simulink model "discreteMod2"  (R2019b)
settings: Solver=VariableStepAuto  StartTime=0.0  StopTime=10.0  RelTol=1e-3
settings Model: Creator=Daniel  LastModifiedBy=Daniel

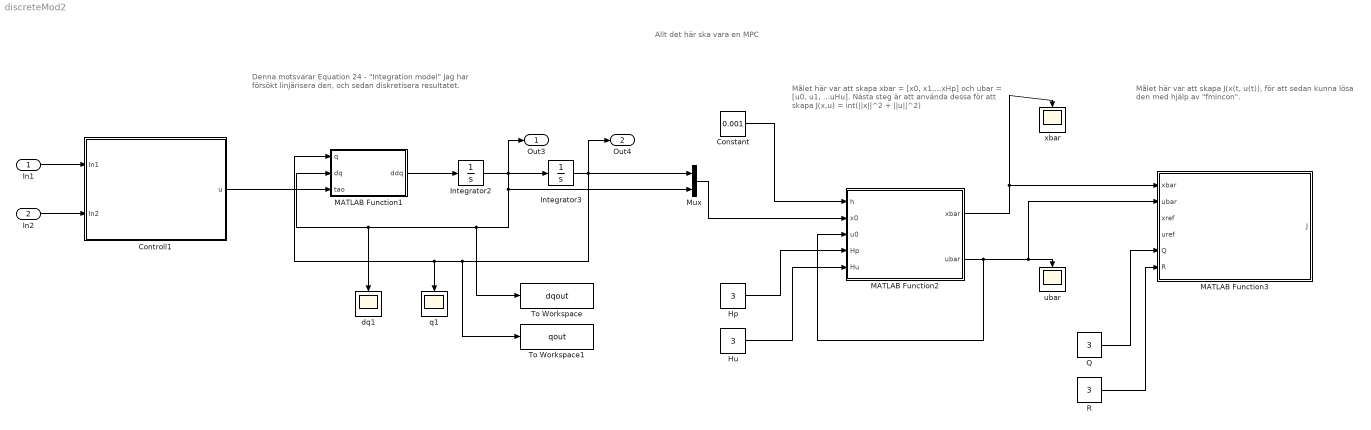
== system discreteMod2 ==
  note: Allt det här ska vara en MPC
  note: Målet här var att skapa J(x(t, u(t)), för att sedan
      | kunna lösa den med hjälp av "fmincon".
  note: Målet här var att skapa xbar = [x0, x1,...xHp]
      | och ubar = [u0, u1, ...uHu].
      | Nästa steg är att använda dessa för att skapa
      | J(x,u) = int(||x||^2 + ||u||^2)
  note: Denna motsvarar
      | Equation 24 - "Integration model"
      | Jag har försökt linjärisera den, och sedan
      | diskretisera resultatet.
  In1 : Inport
  In2 : Inport  Port=2
  Constant : Constant  Value=0.001
  Controll1 : Subsystem
  "Hp " : Constant  Value=3
  "Hu " : Constant  Value=3
  Integrator2 : Integrator  InitialCondition=[0;pi/6]
  Integrator3 : Integrator  InitialCondition=[0;0]
  MATLAB Function1 : MATLAB Function  TreatAsAtomicUnit=on
  MATLAB Function2 : MATLAB Function  TreatAsAtomicUnit=on
  MATLAB Function3 : MATLAB Function  TreatAsAtomicUnit=on
  Mux : Mux  Inputs=2
  Q : Constant  Value=3
  R : Constant  Value=3
  To Workspace : ToWorkspace  VariableName=dqout  SaveFormat=Timeseries  SampleTime=-1
  To Workspace1 : ToWorkspace  VariableName=qout  SampleTime=-1
  dq1 : Scope
  q1 : Scope
  ubar : Scope
  xbar : Scope
  Out3 : Outport
  Out4 : Outport  Port=2
  wires:
  R/1 -> MATLAB Function3/6(R)
  Q/1 -> MATLAB Function3/5(Q)
  MATLAB Function2/2(ubar) -> MATLAB Function2/3(u0), MATLAB Function3/2(ubar), ubar/1
  Mux/1 -> MATLAB Function2/2(x0)
  "Hu "/1 -> MATLAB Function2/5(Hu)
  MATLAB Function2/1(xbar) -> MATLAB Function3/1(xbar), xbar/1
  "Hp "/1 -> MATLAB Function2/4(Hp)
  Constant/1 -> MATLAB Function2/1(h)
  In2/1 -> Controll1/2(In2)
  Controll1/1(u) -> MATLAB Function1/3(tao)
  In1/1 -> Controll1/1(In1)
  Integrator3/1 -> Mux/1, To Workspace1/1, MATLAB Function1/1(q), q1/1, Out4/1
  MATLAB Function1/1(ddq) -> Integrator2/1
  Integrator2/1 -> Mux/2, To Workspace/1, MATLAB Function1/2(dq), dq1/1, Integrator3/1, Out3/1

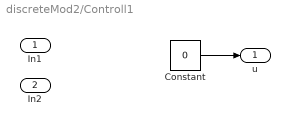
== system discreteMod2/Controll1 ==
  In1 : Inport
  In2 : Inport  Port=2
  Constant : Constant  Value=0
  u : Outport
  wires:
  Constant/1 -> u/1

== matlab function discreteMod2/MATLAB Function1 ==
  data: q input; ddq output; dq input; tao input
function  ddq  = testing(q,dq,tao)
%% q= [phi, theta],   dq = [dphi, dtheta]
tao2=[0;tao];
phi = q(1,1);
theta = q(2,1);
dphi = dq(1,1);
dtheta = dq(2,1);
%Given parameters - "competition.pdf"
la  = 75*10^-3;       %[m]      - Length of arm
r  = 43*10^-3;       %[m]      - Base radius
lp  = 31.5*10^-3;     %[m]      - Length of pendulum
J  = 125*10^-6;      %[kgm^2]  - Base moment of inertia
g  = 9.8;            %[m/s^2]  - Gravity
Jc = 2.55*10^-6;     %[kgm^2]  - Moment of inertia of pendulum around c.o.m
M  = 5.44*10^-3;     %[kg]     - Mass of pendulum point mass
Jp = 7.95*10^-6;     %[kgm^2]  - Moment of inertia of pend around pivot

%Still unknown - Try to guess these as a first step
ma = 10*10^-3;       %[kg] - Mass of arm       - Try 10g
mp = 5*10^-3;        %[kg] - Mass of pendulum  - Try 5g

%Equation (17)
global alpha beta gamma delta;
alpha   = J + (M + (1/3)*ma + mp)*la^2;
beta    = (M + (1/3)*mp)*lp^2;
gamma   = (M + (1/2)*mp)*la*lp;
delta   = (M + (1/2)*mp)*g*lp;

D = [(alpha + beta*sin(theta)^2),(gamma*cos(theta));(gamma*cos(theta)),(beta)];
C = [(beta*cos(theta)*sin(theta)*dtheta),(beta*cos(theta)*sin(theta)*dphi - gamma*sin(theta)*dtheta);(-beta*cos(theta)*sin(theta)*dphi),(0)];
G = [0;-delta*sin(theta)];

% ddq = inv(D)*(tao2 - C*dq - G);
ddq = D\(tao2 - C*dq - G);
end

== matlab function discreteMod2/MATLAB Function2 ==
  data: h input; x0 input; u0 input; xbar output [0..4*Hp]; ubar output; Hp input; Hu input
function [xbar, ubar] = createBars(h, x0, u0, Hp, Hu)
%Input vector xk = [phi_k, dphi_k, theta_k, dtheta_k], and time step h;
%Output vector xk1 = [phi_{k+1}, dphi_{k+1}, theta_{k+1}, dtheta_{k+1}];

%x = [phi, dphi, theta, dtheta]';    %This is the most recent x (x_k)
% x changed to x=[phi,theta,dphi,dtheta]

if (length(x0) < 4*Hp)
    xbar = zeros(4*Hp,1);
    xbar(1:4) = x0;
else
    xbar = x0;      
end

if (length(u0) < 2*Hu)
    ubar = zeros(2*Hu,1);
    ubar(1:2) = u0;
else
    ubar = u0;
end


%%
% D = [(alpha + beta*sin(theta)^2),(gamma*cos(theta));(gamma*cos(theta)),(beta)];
% C = [(beta*cos(theta)*sin(theta)*dtheta),(beta*cos(theta)*sin(theta)*dphi - gamma*sin(theta)*dtheta);(-beta*cos(theta)*sin(theta)*dphi),(0)];
% G = [0;-delta*sin(theta)];
% 
% % Full model continuous, kommer antagligen vara
% % för resurskrävande att uppdatera matriserna mellan varje iteration.
% dAc = D\(-C -G./x0(3:4));
% dBc = D\[1;1];
% Cc =[0,0];
% Dc =[0];
% Hd = ss(dAc,dBc,Cc,Dc,h);
% dAd = Hd.A;
% dBd = Hd.B;

for i = 2:Hp
    xbar((i*4-3):(i*4-2)) = xbar((i-1)*4-3:(i-1)*4-2) + h*(xbar((i-1)*4-1:(i-1)*4));
    
    theta=xbar((i-1)*4-2,1);
    dphi=xbar((i-1)*4-1,1);
    dtheta=xbar((i-1)*4,1);
    D = [(alpha + beta*sin(theta)^2),(gamma*cos(theta));(gamma*cos(theta)),(beta)];
    C = [(beta*cos(theta)*sin(theta)*dtheta),(beta*cos(theta)*sin(theta)*dphi - gamma*sin(theta)*dtheta);(-beta*cos(theta)*sin(theta)*dphi),(0)];
    G = [0;-delta*sin(theta)];
    ddq = D\(-C -G./xbar((i-1)*4-1:(i-1)*4));
    xbar((i*4-1):(i*4)) = xbar((i-1)*4-1:(i-1)*4) + h*(ddq*xbar((i-1)*4-1:(i-1)*4) + D\ubar((i-1)*2-1:(i-1)*2));
end
%%
% Om vi ska ha en linjära diskreta matris A och B, kan vi antingen använda dAd och dBd som
% är baserad på x0 och u0. Det kanske är för resurskrävande att beräkna
% nya ddq varje iteration. Stegen är inte så långa, så det kanske inte
% hinner bli ett så stort fel över Hp. Eller så kan vi fråga marcus om det
% finns en annan approximation vi kan använda.

Ahp = zeros(4*Hp,4*Hp);
Bhu = zeros(4*Hu,2*Hu);
for i = 1:Hp
    Ahp((4*i-3):(4*i), 1:4) = (1+h*A)^i;        %AHp stämmer nog
end
Brow = zeros(4, 2*Hu);
Brow(1:4, 1:2) = h*B;
Bhu(1:4,:) = Brow;
for j = 2:Hu
    Brow = circshift(Brow',2)';
    Brow(1:4,1:2) = (h*B'*(1+h*A)^(j-1))';
    Bhu(4*j-3:4*j, :) = Brow;
end

xk1 = Ahp(1:4,:)*xbar + Bhu(1:4,:)*ubar;
xbar(1:4,1) = x0(1:4);
xbar = circshift(xbar, 4);
xbar(1:4,1) = xk1(1:4)';
ubar(1:2, 1) = u0(1:2);
ubar = circshift(ubar,2);
%Hur ska ubar uppdateras?

end

== matlab function discreteMod2/MATLAB Function3 ==
  data: xbar input; J output; ubar input; xref input; uref input; Q input; R input
function J  = formJacobian(xbar, ubar, xref, uref, Q, R)
%Try to form the Jacobian defined as J(x,u) = int{||x||^2 + ||u||^2}

%1) Skapa QORO
%2) Multiplicera [(xbar-xbar^r);(ubar-ubar^r))]'*QORO*[xbar-xbar^r] för att få ||x||^2
x = [xbar; ubar];
xr = [xref; uref];
Qmat = Q*eye(length(xbar));
Rmat = R*eye(length(ubar));
QORO = zeros(length(xbar)+length(ubar));
QORO(1:length(xbar),1:length(xbar)) = Qmat;
QORO(length(xbar)+1:end, length(xbar)+1:end) = Rmat;

J = (x-xr)'*QORO*(x-xr);

end
